simulink model "Modulation_cosim"  (Simulink 6.0)
settings: Solver=ode45  StartTime=0.0  StopTime=10.0  RelTol=1e-3
libraries: aldec_ahdl x5
settings Model: LastModifiedBy=arekg
settings DataIOCC: SignalLoggingName=sigsOut
settings DebuggingCC: SolverPrmCheckMsg=none
settings HardwareCC: TargetUnknown=on
settings GRTTargetCC: ModelReferenceCompliant=off  MatFileLogging=off

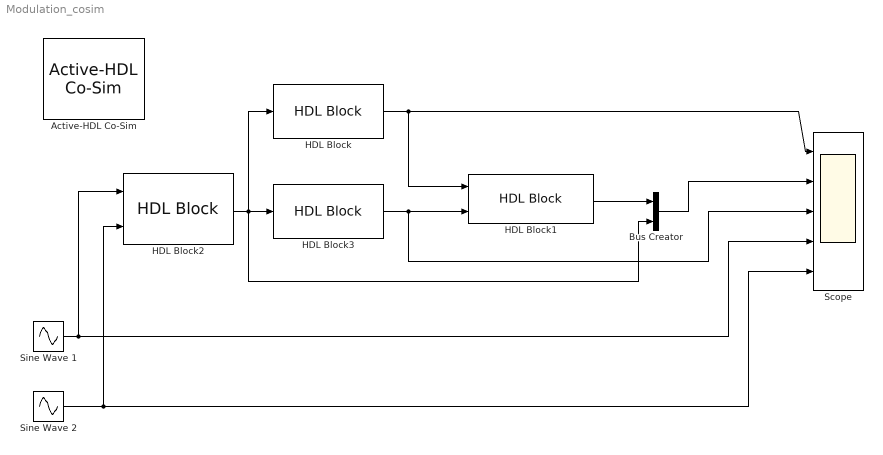
== system Modulation_cosim ==
  Active-HDL Co-Sim : aldec_ahdl/Active-HDL Co-Sim  b_type=0  sys_period=1/20  dbg=off  quit_en=off  gen_tb=off  tb_fn=mlab_post_tb.log
  Bus Creator : BusCreator  DialogController=Simulink.DDGSource_Bus  Inputs=2
  HDL Block : aldec_ahdl/HDL Block  module_m=m_abs_beh  b_type=0  sample=1/20  mode=Enabled  dbg=off
  HDL Block1 : aldec_ahdl/HDL Block  module_m=mult1_beh  b_type=0  sample=1/20  mode=Enabled  dbg=off
  HDL Block2 : aldec_ahdl/HDL Block  module_m=mult_beh  b_type=0  sample=1/20  mode=Enabled  dbg=off
  HDL Block3 : aldec_ahdl/HDL Block  module_m=sign_beh  b_type=0  sample=1/20  mode=Enabled  dbg=off
  Scope : Scope  NumInputPorts=5
      settings: YMin=-1~-40~-2~-1~-1.5  YMax=40~40~2~40~1.5
  Sine Wave 1 : Sin  Amplitude=18  Bias=20  Frequency=0.5*pi  Phase=pi/1.3  SampleTime=1/10
  Sine Wave 2 : Sin  Amplitude=0.9  Frequency=pi/0.4  Phase=pi  SampleTime=1/20
  wires:
  HDL Block/1 -> Scope/1, HDL Block1/1
  Sine Wave 1/1 -> Scope/4, HDL Block2/1
  Sine Wave 2/1 -> Scope/5, HDL Block2/2
  HDL Block2/1 -> Bus Creator/2, HDL Block/1, HDL Block3/1
  HDL Block3/1 -> Scope/3, HDL Block1/2
  HDL Block1/1 -> Bus Creator/1
  Bus Creator/1 -> Scope/2
